simulink model "ctrl_voltage_v17b"  (R2017b)
settings: Solver=FixedStepDiscrete  StartTime=0.0  StopTime=2  FixedStep=Ts_Power  MaxStep=1e-4  RelTol=1e-3
InitFcn:
  | run ctrl_voltage_ini_v17b;
values from neighbouring files (symbols this model uses):
  C = 1e-6    (= 1e-06)    [ctrl_voltage_ini.m]    (also in ctrl_voltage_ini_v17b.m)
  L_t = 1.25e-3    (= 0.00125)    [ctrl_voltage_ini.m]    (also in ctrl_voltage_ini_v17b.m)
  omega = 2*pi*50    (= 314.159265359)    [ctrl_voltage_ini.m]    (also in ctrl_voltage_ini_v17b.m)
  params = [R_t;L_t;R_s;L_s;K_p;K_i;C;K_pv;K_iv]    [ctrl_voltage_ini.m]    (also in ctrl_voltage_ini_v17b.m)
  R_d = 20    [ctrl_voltage_ini.m]    (also in ctrl_voltage_ini_v17b.m)
  R_L = 10    [ctrl_voltage_ini.m]    (also in ctrl_voltage_ini_v17b.m)
  R_t = L_t*omega/10    (= 0.0392699081699)    [ctrl_voltage_ini.m]    (also in ctrl_voltage_ini_v17b.m)
  Ts_Control = 50e-6    (= 5e-05)    [ctrl_voltage_ini.m]    (also in ctrl_voltage_ini_v17b.m)
  Ts_Power = 50e-6    (= 5e-05)    [ctrl_voltage_ini.m]    (also in ctrl_voltage_ini_v17b.m)
  v_dc = 730    [ctrl_voltage_ini.m]    (also in ctrl_voltage_ini_v17b.m)
undefined symbols (not defined in the file or in its folder): DiscIntNeverNeededParam
libraries: powerlib x11, powerlib_meascontrol x2
settings Model: Creator=manuelbarragan  LastModifiedBy=manuelbarragan

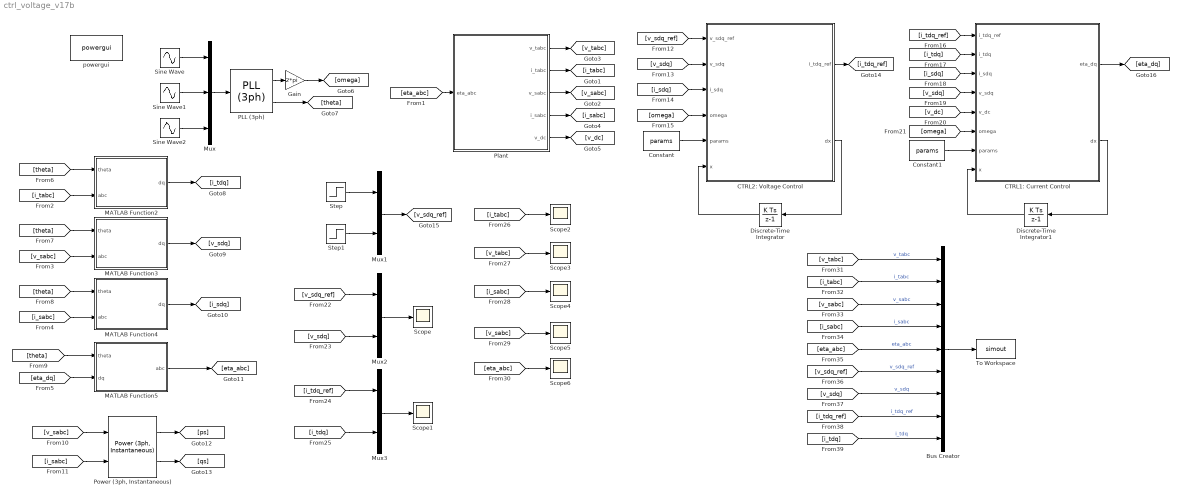
== system ctrl_voltage_v17b ==
  Bus Creator : BusCreator  Inputs=9
  CTRL1: Current Control : MATLAB Function  TreatAsAtomicUnit=on
  CTRL2: Voltage Control : MATLAB Function  TreatAsAtomicUnit=on
  Constant : Constant  Value=params
  Constant1 : Constant  Value=params
  Discrete-Time Integrator : DiscreteIntegrator  InitialCondition=[0;0]  InitialConditionSetting=State (most efficient)  SampleTime=Ts_Control  ICPrevOutput=DiscIntNeverNeededParam  ICPrevScaledInput=DiscIntNeverNeededParam
  Discrete-Time Integrator1 : DiscreteIntegrator  InitialCondition=[0;0]  InitialConditionSetting=State (most efficient)  SampleTime=Ts_Control  ICPrevOutput=DiscIntNeverNeededParam  ICPrevScaledInput=DiscIntNeverNeededParam
  Gain : Gain  Gain=2*pi
  MATLAB Function2 : MATLAB Function  TreatAsAtomicUnit=on
  MATLAB Function3 : MATLAB Function  TreatAsAtomicUnit=on
  MATLAB Function4 : MATLAB Function  TreatAsAtomicUnit=on
  MATLAB Function5 : MATLAB Function  TreatAsAtomicUnit=on
  Mux : Mux  Inputs=3
  Mux1 : Mux  Inputs=2
  Mux2 : Mux  Inputs=2
  Mux3 : Mux  Inputs=2
  PLL (3ph) : powerlib_meascontrol/PLL/PLL (3ph)  Fmin=45  Par_Init=[0, 50]  ParK=[180, 3200, 1]  TcD=1e-4  MaxRateChangeFreq=12  FilterCutOffFreq=25  Ts=Ts_Control  AGC=on
  Plant : Subsystem
  "Power (3ph, Instantaneous)" : powerlib_meascontrol/Measurements/Power (3ph, Instantaneous)
      settings: SourceProductName=Simscape Power Systems
  Scope{,1..6} (7 alike) : Scope
  Sine Wave : Sin  Frequency=omega  SampleTime=Ts_Control
  Sine Wave1 : Sin  Frequency=omega  Phase=-2*pi/3  SampleTime=Ts_Control
  Sine Wave2 : Sin  Frequency=omega  Phase=2*pi/3  SampleTime=Ts_Control
  Step : Step  After=50  SampleTime=0
  Step1 : Step  Time=0.2  After=-230*sqrt(2)  SampleTime=0
  To Workspace : ToWorkspace  VariableName=simout  SaveFormat=Timeseries  SampleTime=-1
  powergui : powerlib/powergui  Priority=1  SimulationMode=Discrete  SampleTime=Ts_Power  frequency=60  Iterations=50  frequencyindice=0  Pbase=100e6  ErrMax=1e-4  UnitsV=kV  UnitsW=MW  buscounter=0  FunctionMessages=off  echomessages=off  EnableUseOfTLC=off  CurrentSourceSwitches=off  DisableSnubberDevices=off  DisableRonSwitches=off  DisableVfSwitches=off  DisplayEquations=off  SolverType=Tustin/Backward Euler (TBE)  Interpol=off  ExternalGateDelay=off  methode=off  Ts=100  x0status=blocks  SPID=on  SwTol=0  HookPort=off  RestoreLinks=warning  ResistiveCurrentMeasurement=off  Frange=[0:2:500]  Ylog=off  Xlog=on  ShowGrid=off  save=off  variable=ZData  structure=0  ZoomFFT=off  StartTime=0.0  cycles=1  DisplayStyle=1  fundamental=60  FreqAxis=off  MaxFrequency=1000  frequencyindicesteady=1  RmsSteady=1  display=off
  wires:
  [eta_abc] -> Plant/1(eta_abc)
  Plant/1(v_tabc) -> [v_tabc]
  Plant/2(i_tabc) -> [i_tabc]
  Plant/5(v_dc) -> [v_dc]
  Plant/4(i_sabc) -> [i_sabc]
  Plant/3(v_sabc) -> [v_sabc]
  [i_tabc] -> MATLAB Function2/2(abc)
  [v_sabc] -> MATLAB Function3/2(abc)
  [i_sabc] -> MATLAB Function4/2(abc)
  [eta_dq] -> MATLAB Function5/2(dq)
  Sine Wave/1 -> Mux/1
  Sine Wave1/1 -> Mux/2
  Sine Wave2/1 -> Mux/3
  Mux/1 -> PLL (3ph)/1
  PLL (3ph)/2 -> [theta]
  PLL (3ph)/1 -> Gain/1
  [theta] -> MATLAB Function2/1(theta)
  [theta] -> MATLAB Function3/1(theta)
  [theta] -> MATLAB Function4/1(theta)
  [theta] -> MATLAB Function5/1(theta)
  MATLAB Function5/1(abc) -> [eta_abc]
  MATLAB Function4/1(dq) -> [i_sdq]
  MATLAB Function3/1(dq) -> [v_sdq]
  MATLAB Function2/1(dq) -> [i_tdq]
  [i_sabc] -> "Power (3ph, Instantaneous)"/2
  [v_sabc] -> "Power (3ph, Instantaneous)"/1
  "Power (3ph, Instantaneous)"/2 -> [qs]
  "Power (3ph, Instantaneous)"/1 -> [ps]
  Gain/1 -> [omega]
  Constant/1 -> CTRL2: Voltage Control/5(params)
  [omega] -> CTRL2: Voltage Control/4(omega)
  [i_sdq] -> CTRL2: Voltage Control/3(i_sdq)
  [v_sdq] -> CTRL2: Voltage Control/2(v_sdq)
  [v_sdq_ref] -> CTRL2: Voltage Control/1(v_sdq_ref)
  CTRL2: Voltage Control/2(dx) -> Discrete-Time Integrator/1
  Discrete-Time Integrator/1 -> CTRL2: Voltage Control/6(x)
  CTRL2: Voltage Control/1(i_tdq_ref) -> [i_tdq_ref]
  [i_tdq_ref] -> CTRL1: Current Control/1(i_tdq_ref)
  [i_tdq] -> CTRL1: Current Control/2(i_tdq)
  [i_sdq] -> CTRL1: Current Control/3(i_sdq)
  [v_sdq] -> CTRL1: Current Control/4(v_sdq)
  [v_dc] -> CTRL1: Current Control/5(v_dc)
  [omega] -> CTRL1: Current Control/6(omega)
  Constant1/1 -> CTRL1: Current Control/7(params)
  CTRL1: Current Control/2(dx) -> Discrete-Time Integrator1/1
  Discrete-Time Integrator1/1 -> CTRL1: Current Control/8(x)
  Step/1 -> Mux1/1
  Step1/1 -> Mux1/2
  Mux1/1 -> [v_sdq_ref]
  [v_sdq_ref] -> Mux2/1
  [v_sdq] -> Mux2/2
  Mux2/1 -> Scope/1
  CTRL1: Current Control/1(eta_dq) -> [eta_dq]
  Mux3/1 -> Scope1/1
  [i_tdq] -> Mux3/2
  [i_tdq_ref] -> Mux3/1
  [i_tabc] -> Scope2/1
  [v_tabc] -> Scope3/1
  [i_sabc] -> Scope4/1
  [v_sabc] -> Scope5/1
  [eta_abc] -> Scope6/1
  [v_tabc] -> Bus Creator/1  "v_tabc"
  [i_tabc] -> Bus Creator/2  "i_tabc"
  [v_sabc] -> Bus Creator/3  "v_sabc"
  [i_sabc] -> Bus Creator/4  "i_sabc"
  [eta_abc] -> Bus Creator/5  "eta_abc"
  [v_sdq_ref] -> Bus Creator/6  "v_sdq_ref"
  [v_sdq] -> Bus Creator/7  "v_sdq"
  [i_tdq_ref] -> Bus Creator/8  "i_tdq_ref"
  [i_tdq] -> Bus Creator/9  "i_tdq"
  Bus Creator/1 -> To Workspace/1

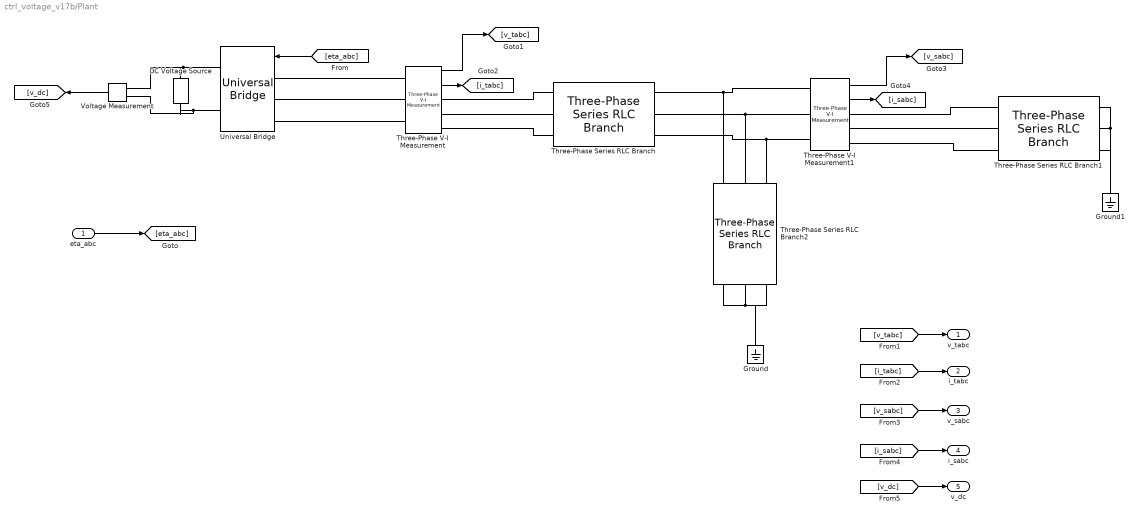
== system ctrl_voltage_v17b/Plant ==
  eta_abc : Inport
  DC Voltage Source : powerlib/Electrical Sources/DC Voltage Source  Amplitude=v_dc  Measurements=None
  Ground : powerlib/Elements/Ground  LConnTagsString=a
  Ground1 : powerlib/Elements/Ground  LConnTagsString=a
  Three-Phase Series RLC Branch : powerlib/Elements/Three-Phase Series RLC Branch  LConnTagsString=A|B|C  RConnTagsString=A|B|C  BranchType=RL  Resistance=R_t  Inductance=L_t  Capacitance=1e-6  Measurements=None
  Three-Phase Series RLC Branch1 : powerlib/Elements/Three-Phase Series RLC Branch  LConnTagsString=A|B|C  RConnTagsString=A|B|C  BranchType=R  Resistance=R_L  Inductance=L_t  Capacitance=1e-6  Measurements=None
  Three-Phase Series RLC Branch2 : powerlib/Elements/Three-Phase Series RLC Branch  LConnTagsString=A|B|C  RConnTagsString=A|B|C  BranchType=RC  Resistance=R_d  Inductance=L_t  Capacitance=C  Measurements=None
  Three-Phase V-I Measurement : powerlib/Measurements/Three-Phase V-I Measurement  VoltageMeasurement=phase-to-ground  SetLabelV=off  LabelV=Vabc  Vpu=off  VpuLL=off  CurrentMeasurement=yes  SetLabelI=off  LabelI=Iabc  Ipu=off  Pbase=100e6  Vbase=500e3  OutputType=Complex  PhasorSimulation=off  PSBequivalent=0
  Three-Phase V-I Measurement1 : powerlib/Measurements/Three-Phase V-I Measurement  VoltageMeasurement=phase-to-ground  SetLabelV=off  LabelV=Vabc  Vpu=off  VpuLL=off  CurrentMeasurement=yes  SetLabelI=off  LabelI=Iabc  Ipu=off  Pbase=100e6  Vbase=500e3  OutputType=Complex  PhasorSimulation=off  PSBequivalent=0
  Universal Bridge : powerlib/Power Electronics/Universal Bridge  Arms=3  SnubberResistance=1e5  SnubberCapacitance=inf  Device=Average-model based VSC  Ron=1e-3  Lon=0  ForwardVoltages="[  0  0  ]"  ForwardVoltage=0  GTOparameters=[ 10e-6 , 20e-6 ]  IGBTparameters=[ 1e-6 , 2e-6 ]  Measurements=None  Measurements_2=None  converterType=Rectifier
  Voltage Measurement : powerlib/Measurements/Voltage Measurement  PhasorSimulation=off  OutputType=Complex  PSBequivalent=0
  v_tabc : Outport
  i_tabc : Outport  Port=2
  v_sabc : Outport  Port=3
  i_sabc : Outport  Port=4
  v_dc : Outport  Port=5
  wires:
  Three-Phase V-I Measurement/2 -> [i_tabc]
  Three-Phase V-I Measurement/1 -> [v_tabc]
  [eta_abc] -> Universal Bridge/1
  Three-Phase V-I Measurement1/1 -> [v_sabc]
  Three-Phase V-I Measurement1/2 -> [i_sabc]
  Voltage Measurement/1 -> [v_dc]
  [v_tabc] -> v_tabc/1
  [i_tabc] -> i_tabc/1
  [v_sabc] -> v_sabc/1
  [i_sabc] -> i_sabc/1
  eta_abc/1 -> [eta_abc]
  [v_dc] -> v_dc/1
  connections:
  Three-Phase Series RLC Branch1/LConn1 -- Three-Phase V-I Measurement1/RConn1
  Three-Phase V-I Measurement1/RConn2 -- Three-Phase Series RLC Branch1/LConn2
  DC Voltage Source/RConn1 -- Voltage Measurement/LConn1 -- Universal Bridge/RConn1
  DC Voltage Source/LConn1 -- Voltage Measurement/LConn2 -- Universal Bridge/RConn2
  Three-Phase Series RLC Branch2/RConn1 -- Ground/LConn1 -- Three-Phase Series RLC Branch2/RConn3 -- Three-Phase Series RLC Branch2/RConn2
  Three-Phase Series RLC Branch1/LConn3 -- Three-Phase V-I Measurement1/RConn3
  Three-Phase Series RLC Branch1/RConn1 -- Ground1/LConn1 -- Three-Phase Series RLC Branch1/RConn3 -- Three-Phase Series RLC Branch1/RConn2
  Three-Phase V-I Measurement/LConn1 -- Universal Bridge/LConn1
  Three-Phase V-I Measurement/LConn2 -- Universal Bridge/LConn2
  Three-Phase V-I Measurement/LConn3 -- Universal Bridge/LConn3
  Three-Phase V-I Measurement/RConn1 -- Three-Phase Series RLC Branch/LConn1
  Three-Phase Series RLC Branch/LConn2 -- Three-Phase V-I Measurement/RConn2
  Three-Phase V-I Measurement/RConn3 -- Three-Phase Series RLC Branch/LConn3
  Three-Phase Series RLC Branch/RConn1 -- Three-Phase Series RLC Branch2/LConn1 -- Three-Phase V-I Measurement1/LConn1
  Three-Phase V-I Measurement1/LConn2 -- Three-Phase Series RLC Branch2/LConn2 -- Three-Phase Series RLC Branch/RConn2
  Three-Phase Series RLC Branch/RConn3 -- Three-Phase Series RLC Branch2/LConn3 -- Three-Phase V-I Measurement1/LConn3

== matlab function ctrl_voltage_v17b/CTRL1: Current Control ==
  data: i_tdq_ref input; i_tdq input; i_sdq input; eta_dq output size=2; v_sdq input; v_dc input; omega input; params input; x input; dx output
function [eta_dq,dx] = ctrl_vsc(i_tdq_ref,i_tdq,i_sdq,v_sdq,v_dc,omega,params,x)

% parameters
R_t = params(1);
L_t = params(2);
K_p = params(5);
K_i = params(6);
C = params(7);

%References
i_td_ref = i_tdq_ref(1);
i_tq_ref = i_tdq_ref(2);

%From transformations
%i_td = i_tdq(1); % If current i_tabc is measured
%i_tq = i_tdq(2);
i_sd = i_sdq(1);
i_sq = i_sdq(2);
v_sd = v_sdq(1);
v_sq = v_sdq(2);
i_td = i_sd - C*omega*v_sq; % If current i_tabc is not measured
i_tq = i_sq + C*omega*v_sd;

% from the integrator to the states
xi_itd = x(1);
xi_itq = x(2);


% auxiliar
e_itd = i_td_ref - i_td;
e_itq = i_tq_ref - i_tq;

% derivatives
dxi_itd = e_itd;
dxi_itq = e_itq;


% auxiliar
u_d = K_p*e_itd + K_i*xi_itd;
u_q = K_p*e_itq + K_i*xi_itq;
L = L_t ;
R = R_t ;

% outputs
eta_d = 2/v_dc*(u_d - L*omega*i_tq + v_sd);
eta_q = 2/v_dc*(u_q + L*omega*i_td + v_sq);
eta_dq = [eta_d ; eta_q];


% from derivatives to the integrator
dx = [dxi_itd;dxi_itq];

== matlab function ctrl_voltage_v17b/CTRL2: Voltage Control ==
  data: v_sdq_ref input; i_tdq_ref output; v_sdq input; i_sdq input; omega input; params input; x input; dx output
function [i_tdq_ref,dx]   = fcn(v_sdq_ref,v_sdq,i_sdq,omega,params,x)

% parameters
C = params(7);
K_pv = params(8);
K_iv = params(9);


%References
v_sd_ref = v_sdq_ref(1);
v_sq_ref = v_sdq_ref(2);

%From transformations
i_sd = i_sdq(1);
i_sq = i_sdq(2);
v_sd = v_sdq(1);
v_sq = v_sdq(2);

% from the integrator to the states
xi_vsd = x(1);
xi_vsq = x(2);

% auxiliar
e_vsd = v_sd_ref - v_sd;
e_vsq = v_sq_ref - v_sq;

% derivatives
dxi_vsd = e_vsd;
dxi_vsq = e_vsq;
dx = [dxi_vsd ; dxi_vsq];

% auxiliar
u_d = K_pv*e_vsd + K_iv*xi_vsd;
u_q = K_pv*e_vsq + K_iv*xi_vsq;

% outputs
i_td_ref=u_d-C*omega*v_sq+i_sd;
i_tq_ref=u_q+C*omega*v_sd+i_sq;

i_tdq_ref = [i_td_ref;i_tq_ref];

== matlab function ctrl_voltage_v17b/MATLAB Function2 ==
  data: theta input size=1; dq output; abc input
function dq  = fcn(theta,abc)
%#codegen

T_p = 2.0/3.0*[[ cos(theta), cos(theta-2.0/3.0*pi), cos(theta+2.0/3.0*pi)];
               [-sin(theta),-sin(theta-2.0/3.0*pi),-sin(theta+2.0/3.0*pi)]];
           
dq=T_p*abc;

== matlab function ctrl_voltage_v17b/MATLAB Function3 ==
  data: theta input size=1; dq output; abc input
function dq  = fcn(theta,abc)
%#codegen

T_p = 2.0/3.0*[[ cos(theta), cos(theta-2.0/3.0*pi), cos(theta+2.0/3.0*pi)];
               [-sin(theta),-sin(theta-2.0/3.0*pi),-sin(theta+2.0/3.0*pi)]];
           
dq=T_p*abc;

== matlab function ctrl_voltage_v17b/MATLAB Function4 ==
  data: theta input size=1; dq output; abc input
function dq  = fcn(theta,abc)
%#codegen

T_p = 2.0/3.0*[[ cos(theta), cos(theta-2.0/3.0*pi), cos(theta+2.0/3.0*pi)];
               [-sin(theta),-sin(theta-2.0/3.0*pi),-sin(theta+2.0/3.0*pi)]];
           
dq=T_p*abc;

== matlab function ctrl_voltage_v17b/MATLAB Function5 ==
  data: theta input size=1; abc output size=3; dq input
function abc  = fcn(theta,dq)
%#codegen

T_p_inv = [[            cos(theta),            -sin(theta)];
           [ cos(theta-2.0/3.0*pi), -sin(theta-2.0/3.0*pi)];
           [ cos(theta+2.0/3.0*pi), -sin(theta+2.0/3.0*pi)]];
           
abc=T_p_inv*dq;
